simulink model "ukupni_filtar_simulink"  (Simulink 7.6)
settings: Solver=ode45  StartTime=0.0  StopTime=15000  MaxStep=1  RelTol=1e-3
libraries: simulink x14
settings Model: Creator=Ogi  LastModifiedBy=Ogi

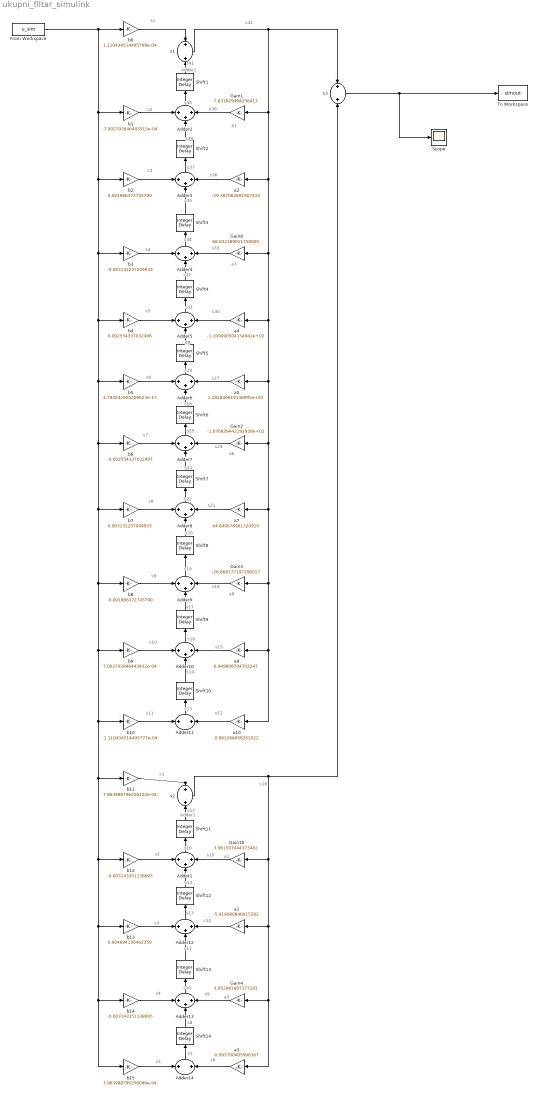
== system ukupni_filtar_simulink ==
  note: a1
  note: a3
  note: a6
  note: a8
  note: Adder1
  note: s1
  note: s2
  note: s3
  note: s4
  note: s5
  note: s6
  note: s7
  note: s8
  note: s9
  note: s10
  note: s11
  note: s12
  note: s13
  note: s14
  note: s15
  note: s16
  note: s17
  note: s18
  note: s19
  note: s20
  note: s21
  note: s22
  note: s23
  note: s24
  note: s26
  note: s27
  note: s28
  note: 29
  note: s30
  note: s31
  note: s32
  note: s33
  note: s34
  note: s35
  note: s36
  note: s37
  note: s38
  note: s39
  note: s40
  note: s41
  note: s42
  note: Adder1
  note: a1
  note: a3
  note: s1
  note: s2
  note: s3
  note: s4
  note: s5
  note: s6
  note: s7
  note: s8
  note: s10
  note: s11
  note: s13
  note: s14
  note: s16
  note: s17
  note: s18
  note: s9
  note: s12
  note: s15
  Adder1 : Sum  Inputs=+++  OutDataTypeStr=fixdt(1, x, y)  RndMeth=Nearest
  Adder{2..10} (9 alike) : Sum  Inputs=+++  OutDataTypeStr=fixdt(1, x , y)  RndMeth=Nearest
  Adder11 : Sum  OutDataTypeStr=fixdt(1, x , y)  RndMeth=Nearest
  Adder12 : Sum  Inputs=+++  OutDataTypeStr=fixdt(1, x, y)  RndMeth=Nearest
  Adder13 : Sum  Inputs=+++  OutDataTypeStr=fixdt(1, x, y)  RndMeth=Nearest
  Adder14 : Sum  OutDataTypeStr=fixdt(1, x, y)  RndMeth=Nearest
  From Workspace : FromWorkspace  VariableName=u_sim
  Gain1 : Gain  Gain=7.831829494256413  ParamDataTypeStr=fixdt(1, j , k)  OutDataTypeStr=fixdt(1, x , y)  RndMeth=Nearest
  Gain10 : Gain  Gain=3.961507444373482  ParamDataTypeStr=fixdt(1, j, k)  OutDataTypeStr=fixdt(1, x, y)  RndMeth=Nearest
  Gain2 : Gain  Gain=-1.076839442192928e+02  ParamDataTypeStr=fixdt(1, j , k)  OutDataTypeStr=fixdt(1, x , y)  RndMeth=Nearest
  Gain3 : Gain  Gain=-26.868177197296017  ParamDataTypeStr=fixdt(1, j , k)  OutDataTypeStr=fixdt(1, x , y)  RndMeth=Nearest
  Gain4 : Gain  Gain=3.952981807177191  ParamDataTypeStr=fixdt(1, j, k)  OutDataTypeStr=fixdt(1, x, y)  RndMeth=Nearest
  Gain8 : Gain  Gain=68.832389011750000  ParamDataTypeStr=fixdt(1, j , k)  OutDataTypeStr=fixdt(1, x , y)  RndMeth=Nearest
  Scope : Scope
  Shift{1..14} (14 alike) : simulink/Discrete/Integer Delay  NumDelays=1  vinit=0.0  samptime=-1
  To Workspace : ToWorkspace  VariableName=simout  SampleTime=-1  SaveFormat=Array
  a1 : Gain  Gain=-5.919080846015582  ParamDataTypeStr=fixdt(1, j, k)  OutDataTypeStr=fixdt(1, x, y)  RndMeth=Nearest
  a10 : Gain  Gain=-0.861266958252022  ParamDataTypeStr=fixdt(1, j , k)  OutDataTypeStr=fixdt(1, x , y)  RndMeth=Nearest
  a2 : Gain  Gain=-29.387062691907410  ParamDataTypeStr=fixdt(1, j , k)  OutDataTypeStr=fixdt(1, x , y)  RndMeth=Nearest
  a3 : Gain  Gain=-0.995700405996367  ParamDataTypeStr=fixdt(1, j, k)  OutDataTypeStr=fixdt(1, x, y)  RndMeth=Nearest
  a4 : Gain  Gain=-1.109490504154942e+02  ParamDataTypeStr=fixdt(1, j , k)  OutDataTypeStr=fixdt(1, x , y)  RndMeth=Nearest
  a5 : Gain  Gain=1.282840619136995e+02  ParamDataTypeStr=fixdt(1, j , k)  OutDataTypeStr=fixdt(1, x , y)  RndMeth=Nearest
  a7 : Gain  Gain=64.840676961320910  ParamDataTypeStr=fixdt(1, j , k)  OutDataTypeStr=fixdt(1, x , y)  RndMeth=Nearest
  a9 : Gain  Gain=6.949806704702247  ParamDataTypeStr=fixdt(1, j , k)  OutDataTypeStr=fixdt(1, x , y)  RndMeth=Nearest
  b0 : Gain  Gain=1.110434514495799e-04  ParamDataTypeStr=fixdt(1, j , k)  OutDataTypeStr=fixdt(1,x,y)  RndMeth=Nearest
  b1 : Gain  Gain=-7.002792846443515e-04  ParamDataTypeStr=fixdt(1, j , k)  OutDataTypeStr=fixdt(1, x , y)  RndMeth=Nearest
  b10 : Gain  Gain=-1.110434514495777e-04  ParamDataTypeStr=fixdt(1, j , k)  OutDataTypeStr=fixdt(1, x , y)  RndMeth=Nearest
  b11 : Gain  Gain=7.963988796256102e-04  ParamDataTypeStr=fixdt(1, j, k)  OutDataTypeStr=fixdt(1, x, y)  RndMeth=Nearest
  b12 : Gain  Gain=-0.003143351138695  ParamDataTypeStr=fixdt(1, j, k)  OutDataTypeStr=fixdt(1, x, y)  RndMeth=Nearest
  b13 : Gain  Gain=0.004694136462350  ParamDataTypeStr=fixdt(1, j, k)  OutDataTypeStr=fixdt(1, x, y)  RndMeth=Nearest
  b14 : Gain  Gain=-0.003143351138695  ParamDataTypeStr=fixdt(1, j, k)  OutDataTypeStr=fixdt(1, x, y)  RndMeth=Nearest
  b15 : Gain  Gain=7.963988796256098e-04  ParamDataTypeStr=fixdt(1, j, k)  OutDataTypeStr=fixdt(1, x, y)  RndMeth=Nearest
  b2 : Gain  Gain=0.001986372745790  ParamDataTypeStr=fixdt(1, j , k)  OutDataTypeStr=fixdt(1, x , y)  RndMeth=Nearest
  b3 : Gain  Gain=-0.003132237049933  ParamDataTypeStr=fixdt(1, j , k)  OutDataTypeStr=fixdt(1, x , y)  RndMeth=Nearest
  b4 : Gain  Gain=0.002554337032496  ParamDataTypeStr=fixdt(1, j , k)  OutDataTypeStr=fixdt(1, x , y)  RndMeth=Nearest
  b5 : Gain  Gain=4.793242905209623e-17  ParamDataTypeStr=fixdt(1, j , k)  OutDataTypeStr=fixdt(1, x , y)  RndMeth=Nearest
  b6 : Gain  Gain=-0.002554337032497  ParamDataTypeStr=fixdt(1, j , k)  OutDataTypeStr=fixdt(1, x , y)  RndMeth=Nearest
  b7 : Gain  Gain=0.003132237049933  ParamDataTypeStr=fixdt(1, j , k)  OutDataTypeStr=fixdt(1, x , y)  RndMeth=Nearest
  b8 : Gain  Gain=-0.001986372745790  ParamDataTypeStr=fixdt(1, j , k)  OutDataTypeStr=fixdt(1, x , y)  RndMeth=Nearest
  b9 : Gain  Gain=7.002792846443432e-04  ParamDataTypeStr=fixdt(1, j , k)  OutDataTypeStr=fixdt(1, x , y)  RndMeth=Nearest
  s1 : Sum  OutDataTypeStr=fixdt(1, x , y)  RndMeth=Nearest
  s2 : Sum  OutDataTypeStr=fixdt(1, x, y)  RndMeth=Nearest
  s3 : Sum  OutDataTypeStr=fixdt(1, 24, 23)  RndMeth=Nearest
  wires:
  Adder3/1 -> Shift2/1
  b1/1 -> Adder2/1
  Shift2/1 -> Adder2/2
  Gain1/1 -> Adder2/3
  Adder2/1 -> Shift1/1
  Shift1/1 -> s1/2
  s1/1 -> Gain1/1, a2/1, Gain8/1, a4/1, Gain2/1, a7/1, Gain3/1, a9/1, a10/1, a5/1, s3/1
  Adder5/1 -> Shift4/1
  b3/1 -> Adder4/1
  Shift4/1 -> Adder4/2
  Gain8/1 -> Adder4/3
  Adder4/1 -> Shift3/1
  a4/1 -> Adder5/3
  Shift3/1 -> Adder3/2
  a2/1 -> Adder3/3
  b2/1 -> Adder3/1
  b4/1 -> Adder5/1
  b0/1 -> s1/1
  From Workspace/1 -> b3/1, b4/1, b7/1, b8/1, b9/1, b10/1, b13/1, b15/1, b14/1, b12/1, b11/1, b6/1, b5/1, b2/1, b1/1, b0/1
  Adder8/1 -> Shift7/1
  b6/1 -> Adder7/1
  Shift7/1 -> Adder7/2
  Gain2/1 -> Adder7/3
  Adder7/1 -> Shift6/1  "s25"
  Shift6/1 -> Adder6/2
  Adder10/1 -> Shift9/1
  b8/1 -> Adder9/1
  Shift9/1 -> Adder9/2
  Gain3/1 -> Adder9/3
  Adder9/1 -> Shift8/1
  a9/1 -> Adder10/3
  Shift8/1 -> Adder8/2
  a7/1 -> Adder8/3
  b7/1 -> Adder8/1
  b9/1 -> Adder10/1
  Adder11/1 -> Shift10/1
  Shift10/1 -> Adder10/2
  a10/1 -> Adder11/2
  b10/1 -> Adder11/1
  b5/1 -> Adder6/1
  a5/1 -> Adder6/3
  Adder6/1 -> Shift5/1
  Shift5/1 -> Adder5/2
  Adder12/1 -> Shift12/1
  b12/1 -> Adder1/1
  Shift12/1 -> Adder1/2
  Gain10/1 -> Adder1/3
  Adder1/1 -> Shift11/1
  Shift11/1 -> s2/2
  s2/1 -> Gain10/1, a1/1, Gain4/1, a3/1, s3/2
  Adder14/1 -> Shift14/1
  b14/1 -> Adder13/1
  Shift14/1 -> Adder13/2
  Gain4/1 -> Adder13/3
  Adder13/1 -> Shift13/1
  a3/1 -> Adder14/2
  Shift13/1 -> Adder12/2
  a1/1 -> Adder12/3
  b13/1 -> Adder12/1
  b15/1 -> Adder14/1
  b11/1 -> s2/1
  s3/1 -> To Workspace/1, Scope/1
